simulink model "SimForces2022a"  (R2022a)
settings: Solver=daessc  StartTime=0.0  StopTime=10  FixedStep=0.001  RelTol=1e-4
values from neighbouring files (symbols this model uses):
  Bc1_V = [0;0;0;0;0;0]    [initializeSimulationGP.m]
  D22F = [0;0;0;0;0;0]    [initializeSimulationGP.m]
  filtDV = init2ndOrderLowPassFilter(35*2*pi,1,controller.dT)    [initializeLowPassFilters.m]
  filtEnc = init2ndOrderLowPassFilter(35*2*pi,1,controller.dT)    [initializeLowPassFilters.m]
undefined symbols (not defined in the file or in its folder): aux, B11_r_B11Tc1, B11_V, B11Ftot, B12_r_B12Tc2, B12_Rot_Tc2, B12_U_Tc2, B12_V, B12Ftot, B31_r_B31B41, B31_V, B31FTot, B32_r_B32B42, B32_Rot_B42, B32_U_B42, B32_V, B32FTot, B41_r_B41Tc1, B41_V, B41FTot, B42_r_B42Tc2, B42_Rot_Tc2, B42_U_Tc2, B42_V, B42FTot, B52_r_B52P32, B52_Rot_P32, B52_U_P32, B52_V, B52Ftot, Bc1_r_Bc1B11, Bc1_r_Bc1B31, Bc1FTot, Bc2_r_Bc2B12, Bc2_r_Bc2B32, Bc2_Rot_B12, Bc2_Rot_B32, Bc2_U_B12, Bc2_U_B32, Bc2_V, Bc2Tot, controller, cyl1, cyl2, D22_V, dq1, dq11, dq12, dq2, dq21, dq22, dx1, dx2, dxt2, fc1, fc1r, fc2, fc2r, fct2, fct2r ... (+61)
libraries: sm_lib x32, nesl_utility x20
(part 2 of 7)

== system SimForces2022a/sbHydraulicManipulatorSimscape/sbLiftLink ==
  note: Resembles an ideal encoder.
  LiftLinkSolid : sm_lib/Body Elements/File Solid  ExtGeomFileName=02_LiftLinkGP.STEP  UnitType=FromFile  ExtGeomFileUnits=m  StepReaderType=OCC  ExportConvexHullGeometry=off  InertiaType=Custom  Mass=80.11363010  MassUnits=kg  CenterOfMass=[0 -0.04248930 0.76135480]  CenterOfMassUnits=m  MomentsOfInertia=[16.37344274 16.11821222 0.72023904]  MomentsOfInertiaUnits=kg*m^2  ProductsOfInertia=[-0.55980815 0 0]  ProductsOfInertiaUnits=kg*m^2  BasedOnType=Mass  Density=7300  DensityUnits=kg/m^3  DoExposeReferenceFrame=off  SerializedFrames=<Frames><Frame><Id>Frame1</Id><Value><Name>F5</Name><Origin><Source>GeometricFeature</Source><FeatureName>cylindrical surface 18</FeatureName></Origin><PrimaryAxis><DefinedDirection>+X</DefinedDirection><Source>ReferenceFrame</Source><SourceDirection>+Z</SourceDirection><FeatureName></FeatureName></PrimaryAxis><SecondaryAxis><DefinedDirection>+Y</DefinedDirection><Source>ReferenceFrame</Source><SourceDirection>+Y</SourceDirection><FeatureName></FeatureName></SecondaryAxis></Value></Frame><Frame><Id>Frame2</Id><Value><Name>F2rot</Name><Origin><Source>GeometricFeature</Source><FeatureName>cylindrical surface 7</FeatureName></Origin><PrimaryAxis><DefinedDirection>+X</DefinedDirection><Source>ReferenceFrame</Source><SourceDirection>+Z</SourceDirection><FeatureName></FeatureName></PrimaryAxis><SecondaryAxis><DefinedDirection>+Y</DefinedDirection><Source>ReferenceFrame</Source><SourceDirection>+Y</SourceDirection><FeatureName></FeatureName></SecondaryAxis></Value></Frame><Frame><Id>Frame3</Id><Value><Name>F3</Name><Origin><Source>GeometricFeature</Source><FeatureName>cylindrical surface 8</FeatureName></Origin><PrimaryAxis><DefinedDirection>+X</DefinedDirection><Source>ReferenceFrame</Source><SourceDirection>+Z</SourceDirection><FeatureName></FeatureName></PrimaryAxis><SecondaryAxis><DefinedDirection>+Y</DefinedDirection><Source>ReferenceFrame</Source><SourceDirection>+Y</SourceDirection><FeatureName></FeatureName></SecondaryAxis></Value></Frame><Frame><Id>Frame4</Id><Value><Name>F4</Name><Origin><Source>GeometricFeature</Source><FeatureName>cylindrical surface 9</FeatureName></Origin><PrimaryAxis><DefinedDirection>+X</DefinedDirection><Source>ReferenceFrame</Source><SourceDirection>+Z</SourceDirection><FeatureName></FeatureName></PrimaryAxis><SecondaryAxis><DefinedDirection>+Y</DefinedDirection><Source>ReferenceFrame</Source><SourceDirection>+Y</SourceDirection><FeatureName></FeatureName></SecondaryAxis></Value></Frame><Frame><Id>Frame5</Id><Value><Name>B11</Name><Origin><Source>GeometricFeature</Source><FeatureName>cylindrical surface 7</FeatureName></Origin><PrimaryAxis><DefinedDirection>+X</DefinedDirection><Source>GeometricFeature</Source><SourceDirection>+Z</SourceDirection><FeatureName>segment 149</FeatureName></PrimaryAxis><SecondaryAxis><DefinedDirection>+Y</DefinedDirection><Source>ReferenceFrame</Source><SourceDirection>+Y</SourceDirection><FeatureName></FeatureName></SecondaryAxis></Value></Frame><Frame><Id>Frame6</Id><Value><Name>Bc2</Name><Origin><Source>GeometricFeature</Source><FeatureName>cylindrical surface 9</FeatureName></Origin><PrimaryAxis><DefinedDirection>+X</DefinedDirection><Source>GeometricFeature</Source><SourceDirection>+Z</SourceDirection><FeatureName>segment 153</FeatureName></PrimaryAxis><SecondaryAxis><DefinedDirection>+Y</DefinedDirection><Source>ReferenceFrame</Source><SourceDirection>+Y</SourceDirection><FeatureName></FeatureName></SecondaryAxis></Value></Frame><Frame><Id>Frame7</Id><Value><Name>Tc1</Name><Origin><Source>GeometricFeature</Source><FeatureName>cylindrical surface 8</FeatureName></Origin><PrimaryAxis><DefinedDirection>+X</DefinedDirection><Source>GeometricFeature</Source><SourceDirection>+Z</SourceDirection><FeatureName>segment 149</FeatureName></PrimaryAxis><SecondaryAxis><DefinedDirection>+Y</DefinedDirection><Source>ReferenceFrame</Source><SourceDirection>+Y</SourceDirection><FeatureName></FeatureName></SecondaryAxis></Value></Frame></Frames>  GraphicType=FromGeometry  MarkerShape=Sphere  MarkerSize=10  GraphicVisPropType=SimpleVisualProperties  GraphicDiffuseColor=[255 192 138]/255  GraphicSpecularColor=[0.5 0.5 0.5 1.0]  GraphicAmbientColor=[0.15 0.15 0.15 1.0]  GraphicEmissiveColor=[0.0 0.0 0.0 1.0]  GraphicShininess=75  GraphicOpacity=1.0
  PS-Simulink Converter : nesl_utility/PS-Simulink Converter  PhysicalDomain=network_engine_domain  SubClassName=ps_output  LeftPortType=input  RightPortType=output  PseudoPeriodic=off  Frequencies=[]  VectorFormat=inherit  Unit=inherit  AffineConversion=off
      settings: SourceProductBaseCode=SS,PW,VE
  Simulink-PS Converter : nesl_utility/Simulink-PS Converter  PhysicalDomain=network_engine_domain  SubClassName=ps_input  LeftPortType=input  RightPortType=output  PseudoPeriodic=off  Frequencies=[]  NoiseDistribution=none  NoiseParameters=[]  Unit=1  AffineConversion=off  FilteringAndDerivatives=filter  SimscapeFilterOrder=2  InputFilterTimeConstant=0.01  UdotUserProvided=0
      settings: SourceProductBaseCode=SS,PW,VE
  Sine Wave : Sin  Amplitude=0.87966  Frequency=0.64555  Phase=-0.12904  SampleTime=0
  theta2Rotation : sm_lib/Joints/Revolute Joint  JointMode=Normal  SenseConstraintForce=off  SenseConstraintForceX=off  SenseConstraintForceY=off  SenseConstraintForceZ=off  SenseConstraintTorque=off  SenseConstraintTorqueX=off  SenseConstraintTorqueY=off  SenseConstraintTorqueZ=off  SenseTotalForce=off  SenseTotalForceX=off  SenseTotalForceY=off  SenseTotalForceZ=off  SenseTotalTorque=off  SenseTotalTorqueX=off  SenseTotalTorqueY=off  SenseTotalTorqueZ=off  CompositeWrenchDir=FollowerOnBase  CompositeWrenchFrame=BaseFrame  EquilibriumPosition=0  EquilibriumPositionUnits=deg  SpringStiffness=0  SpringStiffnessUnits=N*m/deg  DampingCoefficient=0  DampingCoefficientUnits=N*m/(deg/s)  TorqueActuationMode=NoTorque  MotionActuationMode=InputMotion  SensePosition=on  SenseVelocity=off  SenseAcceleration=off  SenseTorqueForce=off  SenseLowerLimitTorqueForce=off  SenseUpperLimitTorqueForce=off  LowerLimitSpecify=off  LowerLimitBound=-90  LowerLimitBoundUnits=deg  LowerLimitStiffness=1e4  LowerLimitStiffnessUnits=N*m/deg  LowerLimitDamping=10  LowerLimitDampingUnits=N*m/(deg/s)  LowerLimitTransitionRegionWidth=0.1  LowerLimitTransitionRegionWidthUnits=deg  UpperLimitSpecify=off  UpperLimitBound=90  UpperLimitBoundUnits=deg  UpperLimitStiffness=1e4  UpperLimitStiffnessUnits=N*m/deg  UpperLimitDamping=10  UpperLimitDampingUnits=N*m/(deg/s)  UpperLimitTransitionRegionWidth=0.1  UpperLimitTransitionRegionWidthUnits=deg  PositionTargetSpecify=on  PositionTargetPriority=High  PositionTargetValue=initVals.theta20  PositionTargetValueUnits=rad  VelocityTargetSpecify=on  VelocityTargetPriority=High  VelocityTargetValue=0  VelocityTargetValueUnits=rad/s
  F4 : PMIOPort  Side=Left
  F5_rot : PMIOPort  Port=2  Side=Left
  F3 : PMIOPort  Port=3  Side=Left
  F2_rot : PMIOPort  Port=4  Side=Right
  Bc2 : PMIOPort  Port=5  Side=Right
  B11 : PMIOPort  Port=6  Side=Right
  Tc1 : PMIOPort  Port=7  Side=Right
  theta2 : Outport
  wires:
  PS-Simulink Converter/1 -> theta2/1
  Sine Wave/1 -> Simulink-PS Converter/1
  connections:
  theta2Rotation/RConn1 -- F5_rot/RConn1
  F2_rot/RConn1 -- LiftLinkSolid/RConn1
  LiftLinkSolid/LConn2 -- F3/RConn1
  F4/RConn1 -- LiftLinkSolid/RConn2
  LiftLinkSolid/LConn1 -- theta2Rotation/LConn1
  LiftLinkSolid/LConn3 -- B11/RConn1
  LiftLinkSolid/LConn4 -- Tc1/RConn1
  Bc2/RConn1 -- LiftLinkSolid/RConn3
  PS-Simulink Converter/LConn1 -- theta2Rotation/RConn2
  Simulink-PS Converter/RConn1 -- theta2Rotation/LConn2

== system SimForces2022a/sbHydraulicManipulatorSimscape/sbPrismaticJointCylinderAndPiston ==
  B52Aux_to_B52 : sm_lib/Frames and Transforms/Rigid Transform  TranslationMethod=None  TranslationStandardOffset=0  TranslationLengthUnit=m  TranslationStandardAxis=+Z  TranslationCartesianOffset=[0 0 0]  TranslationROffset=0  TranslationROffsetUnits=m  TranslationZOffset=0  TranslationZOffsetUnits=m  TranslationThetaOffset=0  TranslationThetaOffsetUnits=deg  RotationMethod=StandardAxis  RotationAngleUnits=deg  RotationStandardAxis=+Y  RotationAngle=-90  RotationArbitraryAxis=[0 0 1]  FollAlignAxisA=+X  BaseAlignAxisA=+Y  FollAlignAxisB=+Y  BaseAlignAxisB=+Z  RotationSequenceAxes=FollowerAxes  RotationSequence=XYX  RotationSequenceAngles=[0 0 0]  RotationSequenceAnglesUnits=deg  RotationMatrix=[1 0 0; 0 1 0; 0 0 1]
  P22p_to_P22pAux : sm_lib/Frames and Transforms/Rigid Transform  TranslationMethod=None  TranslationStandardOffset=0  TranslationLengthUnit=m  TranslationStandardAxis=+Z  TranslationCartesianOffset=[0 0 0]  TranslationROffset=0  TranslationROffsetUnits=m  TranslationZOffset=0  TranslationZOffsetUnits=m  TranslationThetaOffset=0  TranslationThetaOffsetUnits=deg  RotationMethod=StandardAxis  RotationAngleUnits=deg  RotationStandardAxis=+Y  RotationAngle=90  RotationArbitraryAxis=[0 0 1]  FollAlignAxisA=+X  BaseAlignAxisA=+Y  FollAlignAxisB=+Y  BaseAlignAxisB=+Z  RotationSequenceAxes=FollowerAxes  RotationSequence=XYX  RotationSequenceAngles=[0 0 0]  RotationSequenceAnglesUnits=deg  RotationMatrix=[1 0 0; 0 1 0; 0 0 1]
  PS-Sim1 : nesl_utility/PS-Simulink Converter  PhysicalDomain=network_engine_domain  SubClassName=ps_output  LeftPortType=input  RightPortType=output  PseudoPeriodic=off  Frequencies=[]  VectorFormat=1-D array  Unit=inherit  AffineConversion=off
      settings: SourceProductBaseCode=SS,PW,VE
  PS-Sim3 : nesl_utility/PS-Simulink Converter  PhysicalDomain=network_engine_domain  SubClassName=ps_output  LeftPortType=input  RightPortType=output  PseudoPeriodic=off  Frequencies=[]  VectorFormat=1-D array  Unit=inherit  AffineConversion=off
      settings: SourceProductBaseCode=SS,PW,VE
  PrismaticJointCylinder : sm_lib/Body Elements/File Solid  ExtGeomFileName=08_ExtCyl1GP.STEP  UnitType=FromFile  ExtGeomFileUnits=m  StepReaderType=OCC  ExportConvexHullGeometry=off  InertiaType=Custom  Mass=9.26136143  MassUnits=kg  CenterOfMass=[0 0 0.58707478]  CenterOfMassUnits=m  MomentsOfInertia=[1.48398069 1.48387017 0.00662754]  MomentsOfInertiaUnits=kg*m^2  ProductsOfInertia=[0 0 0]  ProductsOfInertiaUnits=kg*m^2  BasedOnType=Density  Density=7850  DensityUnits=kg/m^3  DoExposeReferenceFrame=off  SerializedFrames=<Frames><Frame><Id>Frame1</Id><Value><Name>P22</Name><Origin><Source>GeometricFeature</Source><FeatureName>cylindrical surface 1</FeatureName></Origin><PrimaryAxis><DefinedDirection>+X</DefinedDirection><Source>ReferenceFrame</Source><SourceDirection>-Z</SourceDirection><FeatureName></FeatureName></PrimaryAxis><SecondaryAxis><DefinedDirection>+Y</DefinedDirection><Source>ReferenceFrame</Source><SourceDirection>+Y</SourceDirection><FeatureName></FeatureName></SecondaryAxis></Value></Frame><Frame><Id>Frame2</Id><Value><Name>P22p</Name><Origin><Source>GeometricFeature</Source><FeatureName>planar surface 9</FeatureName></Origin><PrimaryAxis><DefinedDirection>+X</DefinedDirection><Source>ReferenceFrame</Source><SourceDirection>-Z</SourceDirection><FeatureName></FeatureName></PrimaryAxis><SecondaryAxis><DefinedDirection>+Y</DefinedDirection><Source>ReferenceFrame</Source><SourceDirection>+Y</SourceDirection><FeatureName></FeatureName></SecondaryAxis></Value></Frame></Frames>  GraphicType=FromGeometry  MarkerShape=Sphere  MarkerSize=10  GraphicVisPropType=SimpleVisualProperties  GraphicDiffuseColor=[1 1 119]/255  GraphicSpecularColor=[0.5 0.5 0.5 1.0]  GraphicAmbientColor=[0.15 0.15 0.15 1.0]  GraphicEmissiveColor=[0.0 0.0 0.0 1.0]  GraphicShininess=75  GraphicOpacity=1.0
  PrismaticJointPiston : sm_lib/Body Elements/File Solid  ExtGeomFileName=09_ExtPist1GP.STEP  UnitType=FromFile  ExtGeomFileUnits=m  StepReaderType=OCC  ExportConvexHullGeometry=off  InertiaType=Custom  Mass=6.73059863  MassUnits=kg  CenterOfMass=[0 0 0.56802906]  CenterOfMassUnits=m  MomentsOfInertia=[0.91789884 0.91790043 0.00091463]  MomentsOfInertiaUnits=kg*m^2  ProductsOfInertia=[0 0 0]  ProductsOfInertiaUnits=kg*m^2  BasedOnType=Density  Density=7850  DensityUnits=kg/m^3  DoExposeReferenceFrame=off  SerializedFrames=<Frames><Frame><Id>Frame1</Id><Value><Name>B52</Name><Origin><Source>GeometricFeature</Source><FeatureName>planar surface 2</FeatureName></Origin><PrimaryAxis><DefinedDirection>+X</DefinedDirection><Source>ReferenceFrame</Source><SourceDirection>+Z</SourceDirection><FeatureName></FeatureName></PrimaryAxis><SecondaryAxis><DefinedDirection>+Y</DefinedDirection><Source>ReferenceFrame</Source><SourceDirection>-X</SourceDirection><FeatureName></FeatureName></SecondaryAxis></Value></Frame><Frame><Id>Frame2</Id><Value><Name>P32</Name><Origin><Source>GeometricFeature</Source><FeatureName>cylindrical surface 8</FeatureName></Origin><PrimaryAxis><DefinedDirection>+X</DefinedDirection><Source>ReferenceFrame</Source><SourceDirection>+Z</SourceDirection><FeatureName></FeatureName></PrimaryAxis><SecondaryAxis><DefinedDirection>+Y</DefinedDirection><Source>ReferenceFrame</Source><SourceDirection>-X</SourceDirection><FeatureName></FeatureName></SecondaryAxis></Value></Frame></Frames>  GraphicType=FromGeometry  MarkerShape=Sphere  MarkerSize=10  GraphicVisPropType=SimpleVisualProperties  GraphicDiffuseColor=[9 232 232]/255  GraphicSpecularColor=[0.5 0.5 0.5 1.0]  GraphicAmbientColor=[0.15 0.15 0.15 1.0]  GraphicEmissiveColor=[0.0 0.0 0.0 1.0]  GraphicShininess=75  GraphicOpacity=1.0
  Simulink-PS Converter : nesl_utility/Simulink-PS Converter  PhysicalDomain=network_engine_domain  SubClassName=ps_input  LeftPortType=input  RightPortType=output  PseudoPeriodic=off  Frequencies=[]  NoiseDistribution=none  NoiseParameters=[]  Unit=1  AffineConversion=off  FilteringAndDerivatives=filter  SimscapeFilterOrder=2  InputFilterTimeConstant=0.01  UdotUserProvided=0
      settings: SourceProductBaseCode=SS,PW,VE
  Sine Wave : Sin  Amplitude=0.27863  Frequency=0.54472  Phase=0.92559  SampleTime=0
  xt2-joint : sm_lib/Joints/Prismatic Joint  JointMode=Normal  SenseConstraintForce=off  SenseConstraintForceX=off  SenseConstraintForceY=off  SenseConstraintForceZ=off  SenseConstraintTorque=off  SenseConstraintTorqueX=off  SenseConstraintTorqueY=off  SenseConstraintTorqueZ=off  SenseTotalForce=off  SenseTotalForceX=off  SenseTotalForceY=off  SenseTotalForceZ=off  SenseTotalTorque=off  SenseTotalTorqueX=off  SenseTotalTorqueY=off  SenseTotalTorqueZ=off  CompositeWrenchDir=FollowerOnBase  CompositeWrenchFrame=FollowerFrame  EquilibriumPosition=0  EquilibriumPositionUnits=m  SpringStiffness=0  SpringStiffnessUnits=N/m  DampingCoefficient=0  DampingCoefficientUnits=N/(m/s)  TorqueActuationMode=ComputedTorque  MotionActuationMode=InputMotion  SensePosition=on  SenseVelocity=off  SenseAcceleration=off  SenseTorqueForce=on  SenseLowerLimitTorqueForce=off  SenseUpperLimitTorqueForce=off  LowerLimitSpecify=on  LowerLimitBound=0  LowerLimitBoundUnits=m  LowerLimitStiffness=1e6  LowerLimitStiffnessUnits=N/m  LowerLimitDamping=1e3  LowerLimitDampingUnits=N/(m/s)  LowerLimitTransitionRegionWidth=1e-4  LowerLimitTransitionRegionWidthUnits=m  UpperLimitSpecify=on  UpperLimitBound=cylT2.sp  UpperLimitBoundUnits=m  UpperLimitStiffness=1e6  UpperLimitStiffnessUnits=N/m  UpperLimitDamping=1e3  UpperLimitDampingUnits=N/(m/s)  UpperLimitTransitionRegionWidth=1e-4  UpperLimitTransitionRegionWidthUnits=m  PositionTargetSpecify=on  PositionTargetPriority=High  PositionTargetValue=initVals.xt20  PositionTargetValueUnits=m  VelocityTargetSpecify=on  VelocityTargetPriority=High  VelocityTargetValue=0  VelocityTargetValueUnits=m/s
  P22 : PMIOPort  Side=Right
  P32 : PMIOPort  Port=2  Side=Right
  B52 : PMIOPort  Port=3  Side=Right
  fct2 : Outport
  xt2 : Outport  Port=2
  wires:
  PS-Sim3/1 -> fct2/1
  Sine Wave/1 -> Simulink-PS Converter/1
  PS-Sim1/1 -> xt2/1
  connections:
  PrismaticJointPiston/RConn1 -- P32/RConn1
  xt2-joint/RConn1 -- B52Aux_to_B52/LConn1
  B52Aux_to_B52/RConn1 -- B52/RConn1 -- PrismaticJointPiston/LConn1
  P22p_to_P22pAux/RConn1 -- xt2-joint/LConn1
  P22/RConn1 -- PrismaticJointCylinder/LConn1
  P22p_to_P22pAux/LConn1 -- PrismaticJointCylinder/RConn1
  Simulink-PS Converter/RConn1 -- xt2-joint/LConn2
  PS-Sim3/LConn1 -- xt2-joint/RConn3
  PS-Sim1/LConn1 -- xt2-joint/RConn2

== system SimForces2022a/sbHydraulicManipulatorSimscape/sbTilitLink ==
  P22p_to_P22 : sm_lib/Frames and Transforms/Rigid Transform  TranslationMethod=StandardAxis  TranslationStandardOffset=17  TranslationLengthUnit=mm  TranslationStandardAxis=+Z  TranslationCartesianOffset=[0 0 0]  TranslationROffset=0  TranslationROffsetUnits=m  TranslationZOffset=0  TranslationZOffsetUnits=m  TranslationThetaOffset=0  TranslationThetaOffsetUnits=deg  RotationMethod=None  RotationAngleUnits=deg  RotationStandardAxis=+Z  RotationAngle=0.0  RotationArbitraryAxis=[0 0 1]  FollAlignAxisA=+X  BaseAlignAxisA=+Y  FollAlignAxisB=+Y  BaseAlignAxisB=+Z  RotationSequenceAxes=FollowerAxes  RotationSequence=XYX  RotationSequenceAngles=[0 0 0]  RotationSequenceAnglesUnits=deg  RotationMatrix=[1 0 0; 0 1 0; 0 0 1]
  TiltLinkSolid : sm_lib/Body Elements/File Solid  ExtGeomFileName=07_TiltLinkGP.STEP  UnitType=Custom  ExtGeomFileUnits=m  StepReaderType=OCC  ExportConvexHullGeometry=off  InertiaType=Custom  Mass=33.92850233  MassUnits=kg  CenterOfMass=[0.53783811 -0.04670816 0.00002484]  CenterOfMassUnits=m  MomentsOfInertia=[0.31079192 7.19217974 7.40915161]  MomentsOfInertiaUnits=kg*m^2  ProductsOfInertia=[-0.00058487 0.00275052 -0.58280922]  ProductsOfInertiaUnits=kg*m^2  BasedOnType=Density  Density=7300  DensityUnits=kg/m^3  DoExposeReferenceFrame=off  SerializedFrames=<Frames><Frame><Id>Frame1</Id><Value><Name>F5rot</Name><Origin><Source>GeometricFeature</Source><FeatureName>cylindrical surface 12</FeatureName></Origin><PrimaryAxis><DefinedDirection>+Z</DefinedDirection><Source>ReferenceFrame</Source><SourceDirection>+Z</SourceDirection><FeatureName></FeatureName></PrimaryAxis><SecondaryAxis><DefinedDirection>+X</DefinedDirection><Source>ReferenceFrame</Source><SourceDirection>+X</SourceDirection><FeatureName></FeatureName></SecondaryAxis></Value></Frame><Frame><Id>Frame2</Id><Value><Name>F6</Name><Origin><Source>GeometricFeature</Source><FeatureName>cylindrical surface 13</FeatureName></Origin><PrimaryAxis><DefinedDirection>+Z</DefinedDirection><Source>ReferenceFrame</Source><SourceDirection>+Z</SourceDirection><FeatureName></FeatureName></PrimaryAxis><SecondaryAxis><DefinedDirection>+X</DefinedDirection><Source>ReferenceFrame</Source><SourceDirection>+X</SourceDirection><FeatureName></FeatureName></SecondaryAxis></Value></Frame><Frame><Id>Frame3</Id><Value><Name>P22p</Name><Origin><Source>GeometricFeature</Source><FeatureName>circular curve 59</FeatureName></Origin><PrimaryAxis><DefinedDirection>+Y</DefinedDirection><Source>GeometricFeature</Source><SourceDirection>+Z</SourceDirection><FeatureName>segment 349</FeatureName></PrimaryAxis><SecondaryAxis><DefinedDirection>+X</DefinedDirection><Source>ReferenceFrame</Source><SourceDirection>+X</SourceDirection><FeatureName></FeatureName></SecondaryAxis></Value></Frame><Frame><Id>Frame4</Id><Value><Name>Tc2p</Name><Origin><Source>GeometricFeature</Source><FeatureName>cylindrical surface 13</FeatureName></Origin><PrimaryAxis><DefinedDirection>+X</DefinedDirection><Source>GeometricFeature</Source><SourceDirection>+Z</SourceDirection><FeatureName>segment 205</FeatureName></PrimaryAxis><SecondaryAxis><DefinedDirection>+Y</DefinedDirection><Source>ReferenceFrame</Source><SourceDirection>+X</SourceDirection><FeatureName></FeatureName></SecondaryAxis></Value></Frame><Frame><Id>Frame5</Id><Value><Name>B12</Name><Origin><Source>GeometricFeature</Source><FeatureName>cylindrical surface 12</FeatureName></Origin><PrimaryAxis><DefinedDirection>-X</DefinedDirection><Source>GeometricFeature</Source><SourceDirection>+Z</SourceDirection><FeatureName>segment 203</FeatureName></PrimaryAxis><SecondaryAxis><DefinedDirection>+Y</DefinedDirection><Source>ReferenceFrame</Source><SourceDirection>+X</SourceDirection><FeatureName></FeatureName></SecondaryAxis></Value></Frame></Frames>  GraphicType=FromGeometry  MarkerShape=Sphere  MarkerSize=10  GraphicVisPropType=SimpleVisualProperties  GraphicDiffuseColor=[134 134 255]/255  GraphicSpecularColor=[0.5 0.5 0.5 1.0]  GraphicAmbientColor=[0.15 0.15 0.15 1.0]  GraphicEmissiveColor=[0.0 0.0 0.0 1.0]  GraphicShininess=75  GraphicOpacity=1.0
  P22 : PMIOPort  Side=Left
  Tc2 : PMIOPort  Port=2  Side=Left
  B12 : PMIOPort  Port=3  Side=Left
  F6 : PMIOPort  Port=4  Side=Left
  F5_rot : PMIOPort  Port=5  Side=Right
  connections:
  F5_rot/RConn1 -- TiltLinkSolid/LConn1
  F6/RConn1 -- TiltLinkSolid/RConn1
  P22p_to_P22/RConn1 -- P22/RConn1
  P22p_to_P22/LConn1 -- TiltLinkSolid/LConn2
  Tc2/RConn1 -- TiltLinkSolid/RConn2
  B12/RConn1 -- TiltLinkSolid/LConn3

== system SimForces2022a/sbHydraulicManipulatorSimscape/sbTiltCylinderAndTiltPiston ==
  B32Aux : sm_lib/Frames and Transforms/Rigid Transform  TranslationMethod=None  TranslationStandardOffset=0  TranslationLengthUnit=m  TranslationStandardAxis=+Z  TranslationCartesianOffset=[0 0 0]  TranslationROffset=0  TranslationROffsetUnits=m  TranslationZOffset=0  TranslationZOffsetUnits=m  TranslationThetaOffset=0  TranslationThetaOffsetUnits=deg  RotationMethod=StandardAxis  RotationAngleUnits=deg  RotationStandardAxis=+Y  RotationAngle=90  RotationArbitraryAxis=[0 0 1]  FollAlignAxisA=+X  BaseAlignAxisA=+Y  FollAlignAxisB=+Y  BaseAlignAxisB=+Z  RotationSequenceAxes=FollowerAxes  RotationSequence=XYX  RotationSequenceAngles=[0 0 0]  RotationSequenceAnglesUnits=deg  RotationMatrix=[1 0 0; 0 1 0; 0 0 1]
  B42Aux : sm_lib/Frames and Transforms/Rigid Transform  TranslationMethod=None  TranslationStandardOffset=0  TranslationLengthUnit=m  TranslationStandardAxis=+Z  TranslationCartesianOffset=[0 0 0]  TranslationROffset=0  TranslationROffsetUnits=m  TranslationZOffset=0  TranslationZOffsetUnits=m  TranslationThetaOffset=0  TranslationThetaOffsetUnits=deg  RotationMethod=StandardAxis  RotationAngleUnits=deg  RotationStandardAxis=+Y  RotationAngle=-90  RotationArbitraryAxis=[0 0 1]  FollAlignAxisA=+X  BaseAlignAxisA=+Y  FollAlignAxisB=+Y  BaseAlignAxisB=+Z  RotationSequenceAxes=FollowerAxes  RotationSequence=XYX  RotationSequenceAngles=[0 0 0]  RotationSequenceAnglesUnits=deg  RotationMatrix=[1 0 0; 0 1 0; 0 0 1]
  PS-Sim2 : nesl_utility/PS-Simulink Converter  PhysicalDomain=network_engine_domain  SubClassName=ps_output  LeftPortType=input  RightPortType=output  PseudoPeriodic=off  Frequencies=[]  VectorFormat=1-D array  Unit=inherit  AffineConversion=off
      settings: SourceProductBaseCode=SS,PW,VE
  TiltCylinderSolid : sm_lib/Body Elements/File Solid  ExtGeomFileName=05_TiltCylGP.STEP  UnitType=FromFile  ExtGeomFileUnits=m  StepReaderType=OCC  ExportConvexHullGeometry=off  InertiaType=Custom  Mass=17.36281648  MassUnits=kg  CenterOfMass=[0 0.31781210 0]  CenterOfMassUnits=m  MomentsOfInertia=[0.90735702 0.03150902 0.90763033]  MomentsOfInertiaUnits=kg*m^2  ProductsOfInertia=[0 0 0]  ProductsOfInertiaUnits=kg*m^2  BasedOnType=Density  Density=7300  DensityUnits=kg/m^3  DoExposeReferenceFrame=off  SerializedFrames=<Frames><Frame><Id>Frame1</Id><Value><Name>B32</Name><Origin><Source>GeometricFeature</Source><FeatureName>cylindrical surface 11</FeatureName></Origin><PrimaryAxis><DefinedDirection>+X</DefinedDirection><Source>ReferenceFrame</Source><SourceDirection>+Y</SourceDirection><FeatureName></FeatureName></PrimaryAxis><SecondaryAxis><DefinedDirection>+Y</DefinedDirection><Source>ReferenceFrame</Source><SourceDirection>-X</SourceDirection><FeatureName></FeatureName></SecondaryAxis></Value></Frame><Frame><Id>Frame2</Id><Value><Name>B32Aux</Name><Origin><Source>GeometricFeature</Source><FeatureName>planar surface 4</FeatureName></Origin><PrimaryAxis><DefinedDirection>+X</DefinedDirection><Source>ReferenceFrame</Source><SourceDirection>+Y</SourceDirection><FeatureName></FeatureName></PrimaryAxis><SecondaryAxis><DefinedDirection>+Y</DefinedDirection><Source>ReferenceFrame</Source><SourceDirection>-X</SourceDirection><FeatureName></FeatureName></SecondaryAxis></Value></Frame></Frames>  GraphicType=FromGeometry  MarkerShape=Sphere  MarkerSize=10  GraphicVisPropType=SimpleVisualProperties  GraphicDiffuseColor=[1 1 119]/255  GraphicSpecularColor=[0.5 0.5 0.5 1.0]  GraphicAmbientColor=[0.15 0.15 0.15 1.0]  GraphicEmissiveColor=[0.0 0.0 0.0 1.0]  GraphicShininess=75  GraphicOpacity=1.0
  TiltPistonSolid : sm_lib/Body Elements/File Solid  ExtGeomFileName=06_TiltPistGP.STEP  UnitType=FromFile  ExtGeomFileUnits=m  StepReaderType=OCC  ExportConvexHullGeometry=off  InertiaType=Custom  Mass=10.34519231  MassUnits=kg  CenterOfMass=[0 0.32981882 0]  CenterOfMassUnits=m  MomentsOfInertia=[0.55759812 0.00370720 0.55785997]  MomentsOfInertiaUnits=kg*m^2  ProductsOfInertia=[0 0 0]  ProductsOfInertiaUnits=kg*m^2  BasedOnType=Density  Density=7850  DensityUnits=kg/m^3  DoExposeReferenceFrame=off  SerializedFrames=<Frames><Frame><Id>Frame2</Id><Value><Name>B42</Name><Origin><Source>GeometricFeature</Source><FeatureName>planar surface 2</FeatureName></Origin><PrimaryAxis><DefinedDirection>+X</DefinedDirection><Source>ReferenceFrame</Source><SourceDirection>+Y</SourceDirection><FeatureName></FeatureName></PrimaryAxis><SecondaryAxis><DefinedDirection>+Y</DefinedDirection><Source>ReferenceFrame</Source><SourceDirection>-X</SourceDirection><FeatureName></FeatureName></SecondaryAxis></Value></Frame><Frame><Id>Frame3</Id><Value><Name>P11</Name><Origin><Source>GeometricFeature</Source><FeatureName>cylindrical surface 8</FeatureName></Origin><PrimaryAxis><DefinedDirection>+X</DefinedDirection><Source>ReferenceFrame</Source><SourceDirection>+Y</SourceDirection><FeatureName></FeatureName></PrimaryAxis><SecondaryAxis><DefinedDirection>+Y</DefinedDirection><Source>ReferenceFrame</Source><SourceDirection>-X</SourceDirection><FeatureName></FeatureName></SecondaryAxis></Value></Frame></Frames>  GraphicType=FromGeometry  MarkerShape=Sphere  MarkerSize=10  GraphicVisPropType=SimpleVisualProperties  GraphicDiffuseColor=[9 232 232]/255  GraphicSpecularColor=[0.5 0.5 0.5 1.0]  GraphicAmbientColor=[0.15 0.15 0.15 1.0]  GraphicEmissiveColor=[0.0 0.0 0.0 1.0]  GraphicShininess=75  GraphicOpacity=1.0
  q21Rotation : sm_lib/Joints/Revolute Joint  JointMode=Normal  SenseConstraintForce=off  SenseConstraintForceX=off  SenseConstraintForceY=off  SenseConstraintForceZ=off  SenseConstraintTorque=off  SenseConstraintTorqueX=off  SenseConstraintTorqueY=off  SenseConstraintTorqueZ=off  SenseTotalForce=off  SenseTotalForceX=off  SenseTotalForceY=off  SenseTotalForceZ=off  SenseTotalTorque=off  SenseTotalTorqueX=off  SenseTotalTorqueY=off  SenseTotalTorqueZ=off  CompositeWrenchDir=FollowerOnBase  CompositeWrenchFrame=BaseFrame  EquilibriumPosition=0  EquilibriumPositionUnits=rad  SpringStiffness=0  SpringStiffnessUnits=N*m/rad  DampingCoefficient=0  DampingCoefficientUnits=N*m/(rad/s)  TorqueActuationMode=NoTorque  MotionActuationMode=ComputedMotion  SensePosition=off  SenseVelocity=off  SenseAcceleration=off  SenseTorqueForce=off  SenseLowerLimitTorqueForce=off  SenseUpperLimitTorqueForce=off  LowerLimitSpecify=off  LowerLimitBound=-90  LowerLimitBoundUnits=deg  LowerLimitStiffness=1e4  LowerLimitStiffnessUnits=N*m/deg  LowerLimitDamping=10  LowerLimitDampingUnits=N*m/(deg/s)  LowerLimitTransitionRegionWidth=0.1  LowerLimitTransitionRegionWidthUnits=deg  UpperLimitSpecify=off  UpperLimitBound=90  UpperLimitBoundUnits=deg  UpperLimitStiffness=1e4  UpperLimitStiffnessUnits=N*m/deg  UpperLimitDamping=10  UpperLimitDampingUnits=N*m/(deg/s)  UpperLimitTransitionRegionWidth=0.1  UpperLimitTransitionRegionWidthUnits=deg  PositionTargetSpecify=off  PositionTargetPriority=High  PositionTargetValue=0  PositionTargetValueUnits=deg  VelocityTargetSpecify=off  VelocityTargetPriority=High  VelocityTargetValue=0  VelocityTargetValueUnits=deg/s
  q22Rotation : sm_lib/Joints/Revolute Joint  JointMode=Normal  SenseConstraintForce=off  SenseConstraintForceX=off  SenseConstraintForceY=off  SenseConstraintForceZ=off  SenseConstraintTorque=off  SenseConstraintTorqueX=off  SenseConstraintTorqueY=off  SenseConstraintTorqueZ=off  SenseTotalForce=off  SenseTotalForceX=off  SenseTotalForceY=off  SenseTotalForceZ=off  SenseTotalTorque=off  SenseTotalTorqueX=off  SenseTotalTorqueY=off  SenseTotalTorqueZ=off  CompositeWrenchDir=FollowerOnBase  CompositeWrenchFrame=BaseFrame  EquilibriumPosition=0  EquilibriumPositionUnits=rad  SpringStiffness=0  SpringStiffnessUnits=N*m/rad  DampingCoefficient=0  DampingCoefficientUnits=N*m/(rad/s)  TorqueActuationMode=NoTorque  MotionActuationMode=ComputedMotion  SensePosition=off  SenseVelocity=off  SenseAcceleration=off  SenseTorqueForce=off  SenseLowerLimitTorqueForce=off  SenseUpperLimitTorqueForce=off  LowerLimitSpecify=off  LowerLimitBound=-90  LowerLimitBoundUnits=deg  LowerLimitStiffness=1e4  LowerLimitStiffnessUnits=N*m/deg  LowerLimitDamping=10  LowerLimitDampingUnits=N*m/(deg/s)  LowerLimitTransitionRegionWidth=0.1  LowerLimitTransitionRegionWidthUnits=deg  UpperLimitSpecify=off  UpperLimitBound=90  UpperLimitBoundUnits=deg  UpperLimitStiffness=1e4  UpperLimitStiffnessUnits=N*m/deg  UpperLimitDamping=10  UpperLimitDampingUnits=N*m/(deg/s)  UpperLimitTransitionRegionWidth=0.1  UpperLimitTransitionRegionWidthUnits=deg  PositionTargetSpecify=off  PositionTargetPriority=High  PositionTargetValue=0  PositionTargetValueUnits=deg  VelocityTargetSpecify=off  VelocityTargetPriority=High  VelocityTargetValue=0  VelocityTargetValueUnits=deg/s
  x2-translation : sm_lib/Joints/Prismatic Joint  JointMode=Normal  SenseConstraintForce=off  SenseConstraintForceX=off  SenseConstraintForceY=off  SenseConstraintForceZ=off  SenseConstraintTorque=off  SenseConstraintTorqueX=off  SenseConstraintTorqueY=off  SenseConstraintTorqueZ=off  SenseTotalForce=off  SenseTotalForceX=off  SenseTotalForceY=off  SenseTotalForceZ=off  SenseTotalTorque=off  SenseTotalTorqueX=off  SenseTotalTorqueY=off  SenseTotalTorqueZ=off  CompositeWrenchDir=FollowerOnBase  CompositeWrenchFrame=FollowerFrame  EquilibriumPosition=0  EquilibriumPositionUnits=m  SpringStiffness=0  SpringStiffnessUnits=N/m  DampingCoefficient=0  DampingCoefficientUnits=N/(m/s)  TorqueActuationMode=ComputedTorque  MotionActuationMode=ComputedMotion  SensePosition=off  SenseVelocity=off  SenseAcceleration=off  SenseTorqueForce=on  SenseLowerLimitTorqueForce=off  SenseUpperLimitTorqueForce=off  LowerLimitSpecify=on  LowerLimitBound=0  LowerLimitBoundUnits=m  LowerLimitStiffness=1e6  LowerLimitStiffnessUnits=N/m  LowerLimitDamping=1e3  LowerLimitDampingUnits=N/(m/s)  LowerLimitTransitionRegionWidth=1e-4  LowerLimitTransitionRegionWidthUnits=m  UpperLimitSpecify=on  UpperLimitBound=cyl2.sp  UpperLimitBoundUnits=m  UpperLimitStiffness=1e6  UpperLimitStiffnessUnits=N/m  UpperLimitDamping=1e3  UpperLimitDampingUnits=N/(m/s)  UpperLimitTransitionRegionWidth=1e-4  UpperLimitTransitionRegionWidthUnits=m  PositionTargetSpecify=on  PositionTargetPriority=Low  PositionTargetValue=0.3  PositionTargetValueUnits=m  VelocityTargetSpecify=on  VelocityTargetPriority=High  VelocityTargetValue=0  VelocityTargetValueUnits=m/s
  B32 : PMIOPort  Side=Left
  B42 : PMIOPort  Port=2  Side=Left
  F4 : PMIOPort  Port=3  Side=Right
  F6 : PMIOPort  Port=4  Side=Right
  fc2 : Outport
  wires:
  PS-Sim2/1 -> fc2/1
  connections:
  TiltCylinderSolid/RConn1 -- B32Aux/LConn1
  x2-translation/RConn1 -- B42Aux/LConn1
  q21Rotation/RConn1 -- TiltCylinderSolid/LConn1 -- B32/RConn1
  B42/RConn1 -- TiltPistonSolid/LConn1 -- B42Aux/RConn1
  B32Aux/RConn1 -- x2-translation/LConn1
  q21Rotation/LConn1 -- F4/RConn1
  TiltPistonSolid/RConn1 -- q22Rotation/LConn1
  q22Rotation/RConn1 -- F6/RConn1
  PS-Sim2/LConn1 -- x2-translation/RConn2

== system SimForces2022a/sbVDCController/sbAuxiliaryJointAngles ==
  note: For more details on relations in this subsystem, please see the supplementary pdf.
      | In the paper qj angles are assumed known beforehand...
  note: Calculate q1 and q2 from measured theta1 and theta2 angles...
  note: Get inputs...
  note: Process data...
  note: Pass to outputs...
  theta1Filt : Inport
  theta2Filt : Inport  Port=2
  q1Angle : MATLAB Function  TreatAsAtomicUnit=on
  q2Angle : MATLAB Function  TreatAsAtomicUnit=on
  q1 : Outport
  q2 : Outport  Port=2
  wires:
  q2Angle/1(q2) -> [q2]  "q2"
  [q2] -> q2/1  "q2"
  [q1] -> q1/1  "q1"
  q1Angle/1(q1) -> [q1]  "q1"
  [theta1Filt] -> q1Angle/1(theta1Filt)  "theta1Filt"
  [theta2Filt] -> q2Angle/1(theta2Filt)  "theta2Filt"
  theta2Filt/1 -> [theta2Filt]  "theta2Filt"
  theta1Filt/1 -> [theta1Filt]  "theta1Filt"

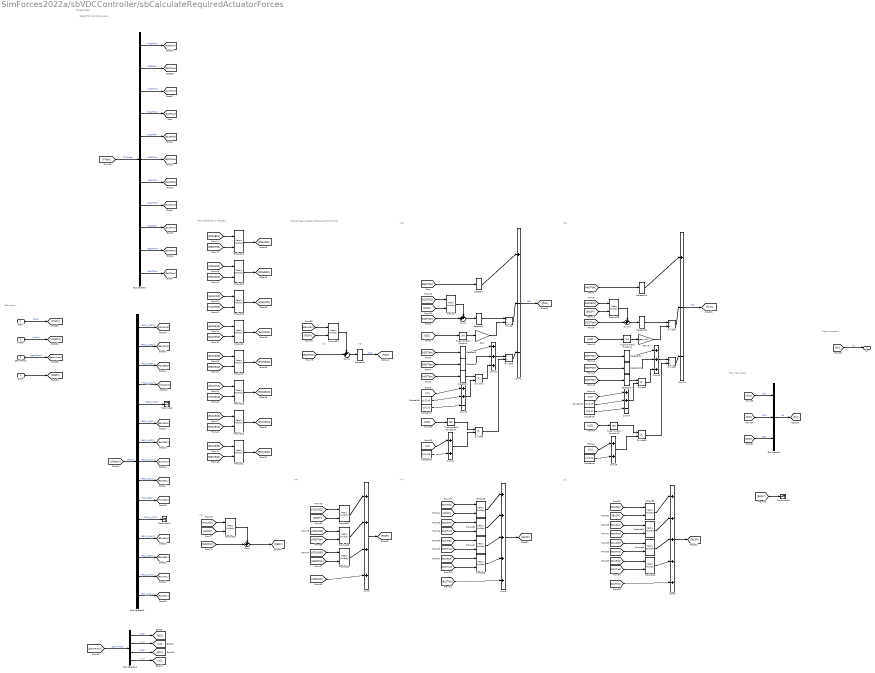
== system SimForces2022a/sbVDCController/sbCalculateRequiredActuatorForces ==
  note: (73)
  note: Get inputs...
  note: Select from existing buses...
  note: Form additional U matrices...
  note: (76)
  note: (76)
  note: (77)
  note: (77)
  note: Extract linear actuator forces per (73) and (76).
  note: Process data...
  note: Form new buses...
  note: Pass to outputs...
  note: (74)
  note: (71)
  note: (72)
  FTotX : Inport
  UMatsX : Inport  Port=2
  geomPropX : Inport  Port=3
  D22F : Inport  Port=4
  Bus Creator1 : BusCreator  Inputs=fc1r,fc2r,fct2r
  Bus Selector : BusSelector  OutputSignals=FTotPS2.P32FTot,FTotPS2.B52Ftot,FTotPS2.P22FTot,FTotRS2.B42FTot,FTotRS2.B12Ftot,FTotRS2.B32FTot,FTotRS2.Bc2Tot,FTotRS1.B41FTot,FTotRS1.B11Ftot,FTotRS1.B31FTot,FTotRS1.Bc1FTot
  Bus Selector1 : BusSelector  OutputSignals=geomPropRS2.q22,geomPropRS2.x2,geomPropRS1.q12,geomPropRS1.x1
  Bus Selector2 : BusSelector  OutputSignals=UMatsPS2.P32_U_D22,UMatsPS2.B52_U_P32,UMatsPS2.P22_U_B52,UMatsRS2.Tc2_U_P22,UMatsRS2.B42_U_Tc2,UMatsRS2.B32_U_B42,UMatsRS2.Bc2_U_B32,UMatsRS2.B12_U_Tc2,UMatsRS2.Bc2_U_B12,UMatsRS1.Tc1_U_Bc2,UMatsRS1.B41_U_Tc1,UMatsRS1.B31_U_B41,UMatsRS1.Bc1_U_B31,UMatsRS1.B11_U_Tc1,UMatsRS1.Bc1_U_B11
  Constant1 : Constant  Value=cyl2.lc
  Constant2 : Constant  Value=cyl1.lc
  Constant3 : Constant  Value=cyl1.x0
  Constant4 : Constant  Value=cyl1.x0
  Constant5 : Constant  Value=cyl2.x0
  Constant6 : Constant  Value=cyl2.x0
  Divide{,5,7,9} (4 alike) : Product  Inputs=*/
  Divide{1,6,8,10} (4 alike) : Product  Inputs=**
  Gain : Gain  Gain=geom.L21
  Gain5 : Gain  Gain=geom.L11
  Product{,1..16,18..23} (23 alike) : Product  Multiplication=Matrix(*)
  Selector : Selector  IndexMode=Zero-based  InputPortWidth=6  IndexOptions=Index vector (dialog)  Indices=[0]  OutputSizes=1
  Selector{1..3,11..13} (6 alike) : Selector  IndexMode=Zero-based  InputPortWidth=6  IndexOptions=Index vector (dialog)  Indices=[5]  OutputSizes=1
  Selector10 : Selector  IndexMode=Zero-based  InputPortWidth=6  IndexOptions=Index vector (dialog)  Indices=[0]  OutputSizes=1
  Selector14 : Selector  IndexMode=Zero-based  InputPortWidth=6  IndexOptions=Index vector (dialog)  Indices=[1]  OutputSizes=1
  Selector4 : Selector  IndexMode=Zero-based  InputPortWidth=6  IndexOptions=Index vector (dialog)  Indices=[1]  OutputSizes=1
  Selector5 : Selector  IndexMode=Zero-based  InputPortWidth=6  IndexOptions=Index vector (dialog)  Indices=[0]  OutputSizes=1
  Sum1 : Sum  Inputs=|+--
  Sum10 : Sum  Inputs=|++-
  Sum11 : Sum  Inputs=|+++
  Sum12 : Sum  Inputs=|++
  Sum13 : Sum  Inputs=|+--
  Sum14 : Sum  Inputs=|++-
  Sum15 : Sum  Inputs=|+++
  Sum16 : Sum  Inputs=|++
  Sum{3..4,7,17} (4 alike) : Sum  Inputs=++|
  Sum2 : Sum  Inputs=|++++
  Sum5 : Sum  Inputs=|+++++
  Sum6 : Sum  Inputs=|+++++
  Terminator : Terminator
  Terminator1 : Terminator
  Terminator3 : Terminator
  Trigonometric Function : Trigonometry
  Trigonometric Function3 : Trigonometry  Operator=tan
  Trigonometric Function4 : Trigonometry
  Trigonometric Function5 : Trigonometry  Operator=tan
  fcr : Outport
  wires:
  [P22UP32] -> Product13/1
  [P32UD22] -> Product13/2
  Product13/1 -> [P22UD22]
  [Bc1Fr] -> Terminator3/1
  [fct2r] -> Bus Creator1/3  "fct2r"
  Selector5/1 -> [fct2r]  "fct2r"
  Sum3/1 -> Selector5/1
  [B52UP32] -> Product22/1
  [P32Fr] -> Product22/2
  Sum7/1 -> [P32Fr]
  Product23/1 -> Sum7/1
  [P32UD22] -> Product23/1
  [D22Fr] -> Product23/2
  [P32FTotr] -> Sum7/2
  Product22/1 -> Sum3/1
  [B52FTotr] -> Sum3/2
  [P22UB52] -> Product19/1
  [P22UP32] -> Product18/1
  Product21/1 -> [P22UP32]
  [B52UP32] -> Product21/2
  [P22UB52] -> Product21/1
  [P22UD22] -> Product20/1
  [D22Fr] -> Product20/2
  [P32FTotr] -> Product18/2
  [B52FTotr] -> Product19/2
  Product20/1 -> Sum2/1
  Product19/1 -> Sum2/3
  [P22FTotr] -> Sum2/4
  Product18/1 -> Sum2/2
  Sum2/1 -> [P22Fr]
  Bus Selector2/2 -> [B52UP32]  "<B52_U_P32>"
  Bus Selector2/3 -> [P22UB52]  "<P22_U_B52>"
  Bus Selector2/1 -> [P32UD22]  "<P32_U_D22>"
  Bus Selector/1 -> [P32FTotr]  "<P32FTot>"
  Bus Selector/2 -> [B52FTotr]  "<B52Ftot>"
  Bus Selector/3 -> [P22FTotr]  "<P22FTot>"
  [fcr] -> fcr/1  "fcr"
  Bus Creator1/1 -> [fcr]  "fcr"
  [B41FTotr] -> Selector10/1
  Gain5/1 -> Divide7/2
  Trigonometric Function4/1 -> Gain5/1
  Selector10/1 -> Sum13/1
  Divide7/1 -> Sum13/2
  Sum13/1 -> [fc1r]  "fc1r"
  [B11FTotr] -> Sum17/2
  Product16/1 -> Sum17/1
  Sum17/1 -> Selector11/1
  [B11UBc2] -> Product16/1
  [Bc2Fr] -> Product16/2
  Selector11/1 -> Divide7/1
  Divide9/1 -> Sum13/3
  Constant4/1 -> Sum16/2
  [x1] -> Sum16/1
  Selector12/1 -> Sum15/1
  Selector13/1 -> Sum15/2
  Divide8/1 -> Sum15/3
  [B31FTotr] -> Selector12/1
  [B41FTotr] -> Selector13/1
  [B41FTotr] -> Selector14/1
  Selector14/1 -> Divide8/1
  Sum14/1 -> Divide8/2
  Constant2/1 -> Sum14/3
  [x1] -> Sum14/1
  Constant3/1 -> Sum14/2
  [q12] -> Trigonometric Function4/1
  Trigonometric Function5/1 -> Divide10/1
  Sum16/1 -> Divide10/2
  Sum15/1 -> Divide9/1
  Divide10/1 -> Divide9/2
  [q12] -> Trigonometric Function5/1
  [q22] -> Trigonometric Function3/1
  Divide6/1 -> Divide5/2
  Sum11/1 -> Divide5/1
  Sum12/1 -> Divide6/2
  Trigonometric Function3/1 -> Divide6/1
  [geomPropX] -> Bus Selector1/1  "geomPropX"
  [UMatsX] -> Bus Selector2/1  "UMatsX"
  [FTotX] -> Bus Selector/1  "FTotXreq"
  D22F/1 -> [D22Fr]
  geomPropX/1 -> [geomPropX]  "geomPropX"
  UMatsX/1 -> [UMatsX]  "UMatsX"
  FTotX/1 -> [FTotX]  "FTotX"
  [q22] -> Trigonometric Function/1
  [fc2r] -> Bus Creator1/2  "fc2r"
  [fc1r] -> Bus Creator1/1  "fc1r"
  Constant5/1 -> Sum10/2
  [x2] -> Sum10/1
  Constant1/1 -> Sum10/3
  Sum10/1 -> Divide1/2
  Selector4/1 -> Divide1/1
  [B42FTotr] -> Selector4/1
  [B42FTotr] -> Selector3/1
  [B32FTotr] -> Selector2/1
  Divide1/1 -> Sum11/3
  Selector3/1 -> Sum11/2
  Selector2/1 -> Sum11/1
  [x2] -> Sum12/1
  Constant6/1 -> Sum12/2
  Divide5/1 -> Sum1/3
  Selector1/1 -> Divide/1
  Product12/1 -> [Bc1UBc2]
  [B11UTc1] -> Product15/1
  [Tc1UBc2] -> Product15/2
  Product15/1 -> [B11UBc2]
  [B11UBc2] -> Product12/2
  [Bc1UB11] -> Product12/1
  [Bc2UB12] -> Product1/1
  [B12UP22] -> Product1/2
  Product14/1 -> [B12UP22]
  [Tc2UP22] -> Product14/2
  [B12UTc2] -> Product14/1
  [B31UB41] -> Product2/2
  [Bc1UB31] -> Product2/1
  Product2/1 -> [Bc1UB41]
  Product1/1 -> [Bc2UP22]
  [Bc1UBc2] -> Product8/1
  [Bc2Fr] -> Product8/2
  Product8/1 -> Sum6/1
  [Bc1FTotr] -> Sum6/5
  Product11/1 -> Sum6/2
  Product9/1 -> Sum6/3
  Product10/1 -> Sum6/4
  [B11FTotr] -> Product10/2
  [Bc1UB11] -> Product10/1
  [B31FTotr] -> Product9/2
  [B41FTotr] -> Product11/2
  [Bc1UB41] -> Product11/1
  [Bc1UB31] -> Product9/1
  Sum6/1 -> [Bc1Fr]
  Sum5/1 -> [Bc2Fr]
  [Bc2UB32] -> Product4/1
  [Bc2UB42] -> Product6/1
  Product7/1 -> [Bc2UB42]
  [Bc2UB32] -> Product7/1
  [B32UB42] -> Product7/2
  [B42FTotr] -> Product6/2
  [B32FTotr] -> Product4/2
  [Bc2UB12] -> Product5/1
  [B12FTotr] -> Product5/2
  Product5/1 -> Sum5/4
  Product4/1 -> Sum5/3
  Product6/1 -> Sum5/2
  [Bc2Totr] -> Sum5/5
  Product3/1 -> Sum5/1
  [P22Fr] -> Product3/2
  [P22Fr] -> Product/2
  [Bc2UP22] -> Product3/1
  [B12UP22] -> Product/1
  Sum4/1 -> Selector1/1
  Product/1 -> Sum4/1
  [B12FTotr] -> Sum4/2
  Bus Selector2/15 -> [Bc1UB11]  "<Bc1_U_B11>"
  Bus Selector2/14 -> [B11UTc1]  "<B11_U_Tc1>"
  Bus Selector2/13 -> [Bc1UB31]  "<Bc1_U_B31>"
  Bus Selector2/12 -> [B31UB41]  "<B31_U_B41>"
  Bus Selector2/11 -> Terminator1/1  "<B41_U_Tc1>"
  Bus Selector2/10 -> [Tc1UBc2]  "<Tc1_U_Bc2>"
  Bus Selector2/9 -> [Bc2UB12]  "<Bc2_U_B12>"
  Bus Selector2/8 -> [B12UTc2]  "<B12_U_Tc2>"
  Bus Selector2/7 -> [Bc2UB32]  "<Bc2_U_B32>"
  Bus Selector2/6 -> [B32UB42]  "<B32_U_B42>"
  Bus Selector2/5 -> Terminator/1  "<B42_U_Tc2>"
  Bus Selector2/4 -> [Tc2UP22]  "<Tc2_U_P22>"
  Sum1/1 -> [fc2r]  "fc2r"
  Divide/1 -> Sum1/2
  Selector/1 -> Sum1/1
  Trigonometric Function/1 -> Gain/1
  Gain/1 -> Divide/2
  Bus Selector1/3 -> [q12]  "<q12>"
  Bus Selector1/4 -> [x1]  "<x1>"
  Bus Selector1/2 -> [x2]  "<x2>"
  Bus Selector1/1 -> [q22]  "<q22>"
  [B42FTotr] -> Selector/1
  Bus Selector/11 -> [Bc1FTotr]  "<Bc1FTot>"
  Bus Selector/10 -> [B31FTotr]  "<B31FTot>"
  Bus Selector/9 -> [B11FTotr]  "<B11Ftot>"
  Bus Selector/8 -> [B41FTotr]  "<B41FTot>"
  Bus Selector/7 -> [Bc2Totr]  "<Bc2Tot>"
  Bus Selector/5 -> [B12FTotr]  "<B12Ftot>"
  Bus Selector/6 -> [B32FTotr]  "<B32FTot>"
  Bus Selector/4 -> [B42FTotr]  "<B42FTot>"

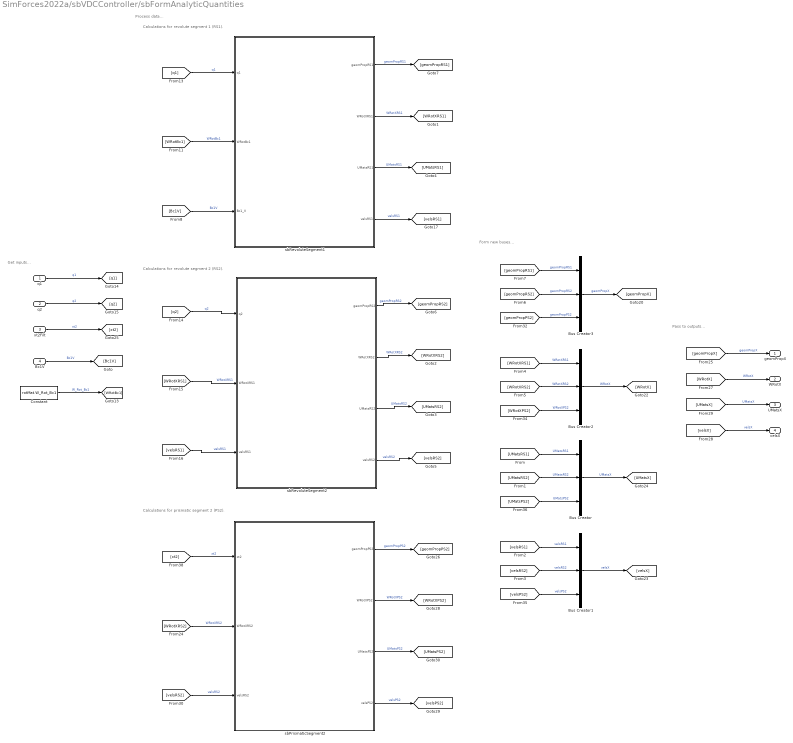
== system SimForces2022a/sbVDCController/sbFormAnalyticQuantities ==
  note: Calculations for prismatic segment 2 (PS2).
  note: Calculations for revolute segment 2 (RS2).
  note: Calculations for revolute segment 1 (RS1).
  note: Get inputs...
  note: Process data...
  note: Form new buses...
  note: Pass to outputs...
  q1 : Inport  Unit=rad  PortDimensions=1
  q2 : Inport  Port=2  Unit=rad  PortDimensions=1
  xt2Filt : Inport  Port=3  Unit=m  PortDimensions=1
  Bc1V : Inport  Port=4
  Bus Creator : BusCreator  Inputs=3
  Bus Creator1 : BusCreator  Inputs=velsRS1,velsRS2,velsPS2
  Bus Creator2 : BusCreator  Inputs=3
  Bus Creator3 : BusCreator  Inputs=3
  Constant : Constant  Value=rotMat.W_Rot_Bc1
  sbPrismaticSegment2 : Subsystem
  sbRevoluteSegment1 : Subsystem
  sbRevoluteSegment2 : Subsystem
  geomPropX : Outport
  WRotX : Outport  Port=2
  UMatsX : Outport  Port=3
  velsX : Outport  Port=4
  wires:
  Bc1V/1 -> [Bc1V]  "Bc1V"
  [velsPS2] -> Bus Creator1/3  "velsPS2"
  [UMatsPS2] -> Bus Creator/3  "UMatsPS2"
  sbPrismaticSegment2/3(UMatsPS2) -> [UMatsPS2]  "UMatsPS2"
  sbPrismaticSegment2/4(velsPS2) -> [velsPS2]  "velsPS2"
  [WRotXPS2] -> Bus Creator2/3  "WRotXPS2"
  sbPrismaticSegment2/2(WRotXPS2) -> [WRotXPS2]  "WRotXPS2"
  [geomPropPS2] -> Bus Creator3/3  "geomPropPS2"
  sbPrismaticSegment2/1(geomPropPS2) -> [geomPropPS2]  "geomPropPS2"
  [velsRS2] -> sbPrismaticSegment2/3(velsRS2)  "velsRS2"
  [WRotXRS2] -> sbPrismaticSegment2/2(WRotXRS2)  "WRotXRS2"
  xt2Filt/1 -> [xt2]  "xt2"
  [UMatsX] -> UMatsX/1  "UMatsX"
  [velsX] -> velsX/1  "velsX"
  [WRotX] -> WRotX/1  "WRotX"
  [geomPropX] -> geomPropX/1  "geomPropX"
  Bus Creator/1 -> [UMatsX]  "UMatsX"
  Bus Creator1/1 -> [velsX]  "velsX"
  Bus Creator2/1 -> [WRotX]  "WRotX"
  Bus Creator3/1 -> [geomPropX]  "geomPropX"
  [geomPropRS1] -> Bus Creator3/1  "geomPropRS1"
  [geomPropRS2] -> Bus Creator3/2  "geomPropRS2"
  [velsRS2] -> Bus Creator1/2  "velsRS2"
  [velsRS1] -> Bus Creator1/1  "velsRS1"
  [UMatsRS1] -> Bus Creator/1  "UMatsRS1"
  [UMatsRS2] -> Bus Creator/2  "UMatsRS2"
  [WRotXRS1] -> Bus Creator2/1  "WRotXRS1"
  [WRotXRS2] -> Bus Creator2/2  "WRotXRS2"
  [q2] -> sbRevoluteSegment2/1(q2)  "q2"
  q2/1 -> [q2]  "q2"
  [q1] -> sbRevoluteSegment1/1(q1)  "q1"
  q1/1 -> [q1]  "q1"
  [Bc1V] -> sbRevoluteSegment1/3(Bc1_V)  "Bc1V"
  [WRotBc1] -> sbRevoluteSegment1/2(WRotBc1)  "WRotBc1"
  Constant/1 -> [WRotBc1]  "W_Rot_Bc1"
  sbRevoluteSegment1/1(geomPropRS1) -> [geomPropRS1]  "geomPropRS1"
  sbRevoluteSegment2/1(geomPropRS2) -> [geomPropRS2]  "geomPropRS2"
  sbRevoluteSegment2/2(WRotXRS2) -> [WRotXRS2]  "WRotXRS2"
  [WRotXRS1] -> sbRevoluteSegment2/2(WRotXRS1)  "WRotXRS1"
  sbRevoluteSegment1/2(WRotXRS1) -> [WRotXRS1]  "WRotXRS1"
  sbRevoluteSegment1/3(UMatsRS1) -> [UMatsRS1]  "UMatsRS1"
  sbRevoluteSegment2/3(UMatsRS2) -> [UMatsRS2]  "UMatsRS2"
  sbRevoluteSegment2/4(velsRS2) -> [velsRS2]  "velsRS2"
  [velsRS1] -> sbRevoluteSegment2/3(velsRS1)  "velsRS1"
  sbRevoluteSegment1/4(velsRS1) -> [velsRS1]  "velsRS1"
  [xt2] -> sbPrismaticSegment2/1(xt2)  "xt2"

== system SimForces2022a/sbVDCController/sbFormTotalRequiredForces ==
  note: Get inputs...
  note: Pass to outputs...
  note: Form new buses...
  note: Process data...
  velsX : Inport
  WRotX : Inport  Port=2
  Bus Creator : BusCreator  Inputs=FTotRS1,FTotRS2,FTotPS2
  sbTotalRequiredForcesPS2 : Subsystem
  sbTotalRequiredForcesRS1 : Subsystem
  sbTotalRequiredForcesRS2 : Subsystem
  FTotX : Outport
  wires:
  [FTotPS2] -> Bus Creator/3  "FTotPS2"
  sbTotalRequiredForcesPS2/1(FTotRS2) -> [FTotPS2]  "FTotPS2"
  [velsX] -> sbTotalRequiredForcesPS2/1(velsX)  "velsX"
  [WRotX] -> sbTotalRequiredForcesPS2/2(WRotX)  "WRotX"
  Bus Creator/1 -> [FTotX]  "FTotX"
  [FTotX] -> FTotX/1  "FTotX"
  [FTotRS1] -> Bus Creator/1  "FTotRS1"
  [FTotRS2] -> Bus Creator/2  "FTotRS2"
  sbTotalRequiredForcesRS1/1(FTotRS1) -> [FTotRS1]  "FTotRS1"
  sbTotalRequiredForcesRS2/1(FTotRS2) -> [FTotRS2]  "FTotRS2"
  [WRotX] -> sbTotalRequiredForcesRS2/2(WRotX)  "WRotX"
  [velsX] -> sbTotalRequiredForcesRS2/1(velsX)  "velsX"
  [velsX] -> sbTotalRequiredForcesRS1/1(velsX)  "velsX"
  WRotX/1 -> [WRotX]  "WRotX"
  velsX/1 -> [velsX]  "velsX"
  [WRotX] -> sbTotalRequiredForcesRS1/2(WRotX)  "WRotX"

== system SimForces2022a/sbVDCController/sbFormAnalyticQuantities/sbPrismaticSegment2 ==
  note: Process data...
  note: Get inputs...
  note: Pass to outputs...
  xt2 : Inport
  WRotXRS2 : Inport  Port=2
  velsRS2 : Inport  Port=3
  sbGeomPropPS2 : Subsystem
  sbPosVecsPS2 : Subsystem
  sbRotMatsPS2 : Subsystem
  sbUMatsPS2 : Subsystem
  sbVelsPS2 : Subsystem
  geomPropPS2 : Outport
  WRotXPS2 : Outport  Port=2
  UMatsPS2 : Outport  Port=3
  velsPS2 : Outport  Port=4
  wires:
  [velsPS2] -> velsPS2/1  "velsPS2"
  sbVelsPS2/1(velsPS2) -> [velsPS2]  "velsPS2"
  [UMatsPS2] -> sbVelsPS2/2(UMatsPS2)  "UMatsPS2"
  [geomPropPS2] -> sbVelsPS2/1(geomPropPS2)  "geomPropPS2"
  [velsRS2] -> sbVelsPS2/3(velsRS2)  "velsRS2"
  [UMatsPS2] -> UMatsPS2/1  "UMatsPS2"
  sbUMatsPS2/1(UMatsPS2) -> [UMatsPS2]  "UMatsPS2"
  [rotMatsPS2] -> sbUMatsPS2/2(rotMatsPS2)  "rotMatsPS2"
  [posVecsPS2] -> sbUMatsPS2/1(posVecsPS2)  "posVecsPS2"
  sbRotMatsPS2/1(rotMatsPS2) -> [rotMatsPS2]  "rotMatsPS2"
  [WRotXPS2] -> WRotXPS2/1  "WRotXPS2"
  [WRotXRS2] -> sbRotMatsPS2/1(WRotXRS2)  "WRotXRS2"
  sbRotMatsPS2/2(WRotXPS2) -> [WRotXPS2]  "WRotXPS2"
  [xt2] -> sbPosVecsPS2/1(xt2)  "xt2"
  sbPosVecsPS2/1(posVecsPS2) -> [posVecsPS2]  "posVecsPS2"
  [xt2] -> sbGeomPropPS2/1(xt2)  "xt2"
  [geomPropPS2] -> geomPropPS2/1  "geomPropPS2"
  WRotXRS2/1 -> [WRotXRS2]  "WRotXRS2"
  velsRS2/1 -> [velsRS2]  "velsRS2"
  xt2/1 -> [xt2]  "xt2"
  sbGeomPropPS2/1(geomPropPS2) -> [geomPropPS2]  "geomPropPS2"

== system SimForces2022a/sbVDCController/sbFormAnalyticQuantities/sbRevoluteSegment1 ==
  note: Form relevant linear/angular velocities per (24) - (31).
  note: Form relevant velocity/force transformation matrices...
  note: Form relevant rotation matrices...
  note: Form relevant position vectors...
  note: Get inputs...
  note: Calculate kinematic quantities (18) - (23) in revolute segment 1 (RS1).
  note: Process data...
  note: Pass to outputs...
  q1 : Inport  Unit=rad
  WRotBc1 : Inport  Port=2
  Bc1_V : Inport  Port=3  PortDimensions=[6 1]
  sbGeomPropRS1 : Subsystem
  sbPosVecsRS1 : Subsystem
  sbRotMatsRS1 : Subsystem
  sbUMatsRS1 : Subsystem
  sbVelsRS1 : Subsystem
  geomPropRS1 : Outport
  WRotXRS1 : Outport  Port=2
  UMatsRS1 : Outport  Port=3
  velsRS1 : Outport  Port=4
  wires:
  [q1] -> sbGeomPropRS1/1(q1)  "q1"
  q1/1 -> [q1]  "q1"
  [WRotXRS1] -> WRotXRS1/1  "WRotXRS1"
  sbRotMatsRS1/2(WRotXRS1) -> [WRotXRS1]  "WRotXRS1"
  [UMatsRS1] -> UMatsRS1/1  "UMatsRS1"
  [WRotBc1] -> sbRotMatsRS1/2(WRotBc1)  "WRotBc1"
  WRotBc1/1 -> [WRotBc1]  "WRotBc1"
  [Bc1V] -> sbVelsRS1/3(Bc1_V)  "Bc1V"
  Bc1_V/1 -> [Bc1V]  "Bc1V"
  [UMatsRS1] -> sbVelsRS1/2(UMatsRS1)  "UMatsRS1"
  sbUMatsRS1/1(UMatsRS1) -> [UMatsRS1]  "UMatsRS1"
  [velsRS1] -> velsRS1/1  "velsRS1"
  sbVelsRS1/1(velsRS1) -> [velsRS1]  "velsRS1"
  [geomPropRS1] -> geomPropRS1/1  "geomPropRS1"
  [posVecsRS1] -> sbUMatsRS1/1(posVecsRS1)  "posVecsRS1"
  sbPosVecsRS1/1(posVecsRS1) -> [posVecsRS1]  "posVecsRS1"
  [rotMatsRS1] -> sbUMatsRS1/2(rotMatsRS1)  "rotMatsRS1"
  sbRotMatsRS1/1(rotMatsRS1) -> [rotMatsRS1]  "rotMatsRS1"
  [geomPropRS1] -> sbVelsRS1/1(geomPropRS1)  "geomPropRS1"
  [geomPropRS1] -> sbRotMatsRS1/1(geomPropRS1)  "geomPropRS1"
  [geomPropRS1] -> sbPosVecsRS1/1(geomPropRS1)  "geomPropRS1"
  sbGeomPropRS1/1(geomPropRS1) -> [geomPropRS1]  "geomPropRS1"
